simulink model "Q_CONTROL_Discret"  (Simulink 8.9)
settings: Solver=FixedStepDiscrete  StartTime=0.0  StopTime=inf  FixedStep=0.002  RelTol=1e-3  EnableMultiTasking=on
values from neighbouring files (symbols this model uses):
  K = place(AD,BD,pDisc)    [model3.m]
  Ts = results(i).Ts    [COMPLATE.m]    (also in model3.m = 0.002; observer_based-control.m = Ts_values(i))
undefined symbols (not defined in the file or in its folder): HIL, K_AMP, K_ENC, K_POT, qc_get_step_size, VMAX_AMP, VMAX_DAC
libraries: quarc_library x7, simulink_extras x4
settings Model: Creator=MLevis  LastModifiedBy=LEGION  SimulationMode=external  ExtModeTrigDuration=50000
settings SolverCC: PositivePriorityOrder=on
settings OptimizationCC: BooleanDataType=off  OptimizeBlockIOStorage=off  BufferReuse=off  GlobalBufferReuse=off  ExpressionFolding=off  ExpressionDepthLimit=2147483647  LocalBlockOutputs=off  InitFltsAndDblsToZero=on  LifeSpan=auto
settings DebuggingCC: SaveWithParameterizedLinksMsg=none  SignalResolutionControl=TryResolveAllWithWarning  MultiTaskDSMMsg=warning  MultiTaskCondExecSysMsg=none
settings RTWCC: Description=QUARC Win64 Target  SystemTargetFile=quarc_win64.tlc  TemplateMakefile=quarc_default_tmf
settings STFCustomTargetCC: TargetPreCompLibLocation=C:\PROGRA~3\QUARC\lib\2017a\win64\release  ConcurrentExecutionCompliant=on  SystemTargetFile=quarc_win64.tlc
settings GRTTargetCC: TargetPreCompLibLocation=C:\PROGRA~3\QUARC\lib\2017a\win64\release  ParMdlRefBuildCompliant=off  CompOptLevelCompliant=off  MatFileLogging=off  CPPClassGenCompliant=off  UseToolchainInfoCompliant=off  ExtMode=on  ExtModeMexFile=quarc_comm

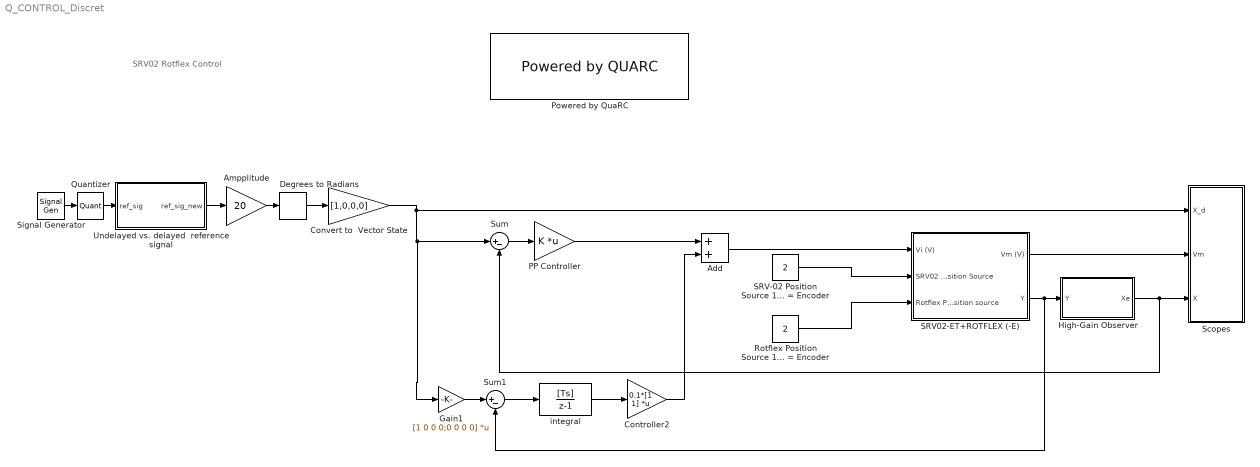
== system Q_CONTROL_Discret ==
  note: SRV02 Rotflex Control
  Add : Sum
  Ampplitude : Gain  Gain=20  SaturateOnIntegerOverflow=on  OutDataTypeStr=Inherit: Same as input  ParamDataTypeStr=Inherit: Same as input
  Controller2 : Gain  Gain=0.1*[1 1]  Multiplication=Matrix(K*u)  SaturateOnIntegerOverflow=on  OutDataTypeStr=Inherit: Same as input  ParamDataTypeStr=Inherit: Same as input
  Convert to  Vector State : Gain  Gain=[1,0,0,0]
  Degrees to Radians : simulink_extras/Transformations/Degrees to Radians
  Gain1 : Gain  Gain=[1 0 0 0;0 0 0 0]  Multiplication=Matrix(K*u)
  High-Gain Observer : Subsystem
  PP Controller : Gain  Gain=K  Multiplication=Matrix(K*u)  SaturateOnIntegerOverflow=on  OutDataTypeStr=Inherit: Same as input  ParamDataTypeStr=Inherit: Same as input
  Powered by QuaRC : quarc_library/Logos/Powered by QUARC
  Quantizer : Quantizer  QuantizationInterval=Ts
  "Rotflex Position Source 1 = Potentiometer, 2 = Encoder" : Constant  Value=2
  "SRV-02 Position Source 1 = Potentiometer, 2 = Encoder" : Constant  Value=2
  SRV02-ET+ROTFLEX (-E) : Subsystem
  Scopes : Subsystem
  Signal Generator : SignalGenerator  WaveForm=square  Frequency=0.3
  Sum : Sum  Inputs=|+-
  Sum1 : Sum  Inputs=|+-
  "Undelayed vs. delayed  reference signal " : Subsystem
  integral : DiscreteTransferFcn  Numerator=[Ts]  Denominator=[1 -1]  SampleTime=Ts
  wires:
  High-Gain Observer/1(Xe) -> Scopes/3(X), Sum/2
  SRV02-ET+ROTFLEX (-E)/2(Y) -> High-Gain Observer/1(Y), Sum1/2
  SRV02-ET+ROTFLEX (-E)/1(Vm (V)) -> Scopes/2(Vm)
  Sum/1 -> PP Controller/1
  Degrees to Radians/1 -> Convert to  Vector State/1
  Convert to  Vector State/1 -> Scopes/1(X_d), Gain1/1, Sum/1
  Ampplitude/1 -> Degrees to Radians/1
  Signal Generator/1 -> Quantizer/1
  "Undelayed vs. delayed  reference signal "/1(ref_sig_new) -> Ampplitude/1
  PP Controller/1 -> Add/1
  "SRV-02 Position Source 1 = Potentiometer, 2 = Encoder"/1 -> SRV02-ET+ROTFLEX (-E)/2(SRV02 Position Source)
  "Rotflex Position Source 1 = Potentiometer, 2 = Encoder"/1 -> SRV02-ET+ROTFLEX (-E)/3(Rotflex Position source)
  Quantizer/1 -> "Undelayed vs. delayed  reference signal "/1(ref_sig)
  Gain1/1 -> Sum1/1
  Sum1/1 -> integral/1
  integral/1 -> Controller2/1
  Add/1 -> SRV02-ET+ROTFLEX (-E)/1(Vi (V))
  Controller2/1 -> Add/2

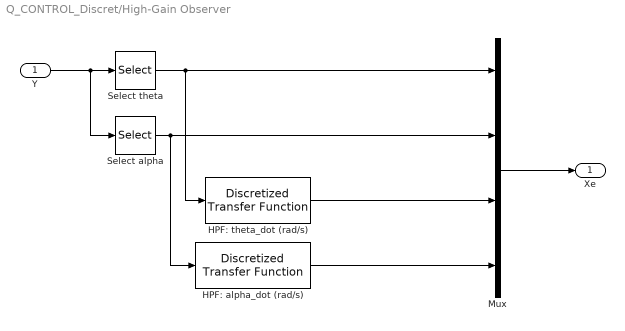
== system Q_CONTROL_Discret/High-Gain Observer ==
  Y : Inport  SampleTime=Ts
  HPF: alpha_dot (rad/s) : quarc_library/Discrete/Discretized Transfer Function  num=[150 0]  den=[1 150]  method=tustin  Ts=qc_get_step_size
  HPF: theta_dot (rad/s) : quarc_library/Discrete/Discretized Transfer Function  num=[150 0]  den=[1 150]  method=tustin  Ts=qc_get_step_size
  Mux : Mux
  Select alpha : Selector  InputPortWidth=2  IndexOptions=Index vector (dialog)  Indices=2  OutputSizes=1
  Select theta : Selector  InputPortWidth=2  IndexOptions=Index vector (dialog)  Indices=1  OutputSizes=1
  Xe : Outport  SampleTime=Ts
  wires:
  HPF: alpha_dot (rad/s)/1 -> Mux/4
  Select theta/1 -> HPF: theta_dot (rad/s)/1, Mux/1
  HPF: theta_dot (rad/s)/1 -> Mux/3
  Y/1 -> Select theta/1, Select alpha/1
  Mux/1 -> Xe/1
  Select alpha/1 -> HPF: alpha_dot (rad/s)/1, Mux/2

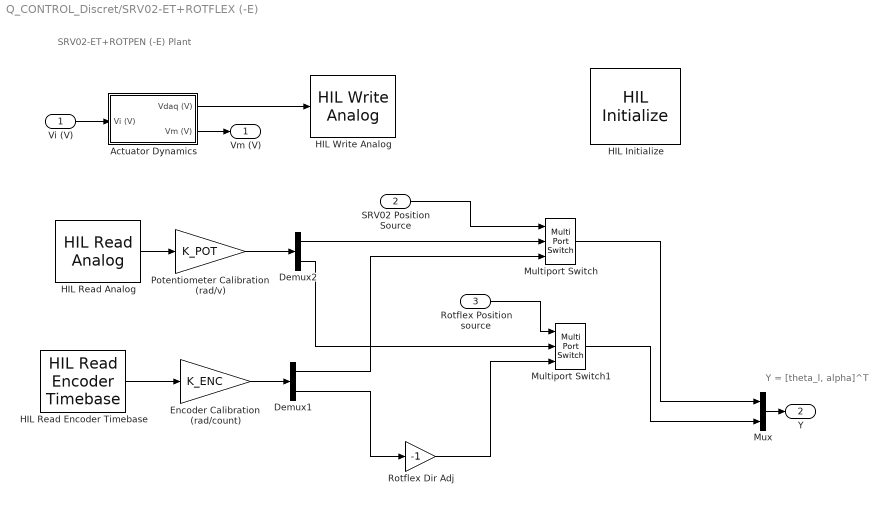
== system Q_CONTROL_Discret/SRV02-ET+ROTFLEX (-E) ==
  note: Y = [theta_l, alpha]^T
  note: SRV02-ET+ROTPEN (-E) Plant
  Vi (V) : Inport  SampleTime=Ts
  SRV02 Position Source : Inport  Port=2  SampleTime=Ts
  Rotflex Position source : Inport  Port=3  SampleTime=Ts
  Actuator Dynamics : Subsystem
  Demux1 : Demux  Outputs=2
  Demux2 : Demux  Outputs=2
  Encoder Calibration  (rad/count) : Gain  Gain=K_ENC  SaturateOnIntegerOverflow=on  OutDataTypeStr=Inherit: Same as input  ParamDataTypeStr=Inherit: Same as input
  HIL Initialize : quarc_library/Data Acquisition/Generic/Configuration/HIL Initialize  object_name=HIL-1  board_type=q2_usb  board_number=0  board_options=d0=digital;d1=digital;led=auto;update_rate=normal;decimation=1  exclusive=off  active=on  hardware_clocks=[0]  clock_modes=[]  initial_clock_frequencies=[]  set_clock_params_at_start=off  set_clock_params_at_switch_in=off  set_clock_frequencies_at_start=off  set_clock_frequencies_at_switch_in=off  analog_input_channels=[0:1]  analog_input_configurations=[]  analog_input_maximums=10  analog_input_minimums=-10  set_analog_input_params_at_start=on  set_analog_input_params_at_switch_in=off  analog_output_channels=[0:1]  analog_output_maximums=10  analog_output_minimums=-10  initial_analog_outputs=[0]  final_analog_outputs=[0]  watchdog_analog_outputs=0  set_analog_output_params_at_start=on  set_analog_output_params_at_switch_in=off  set_analog_outputs_at_start=on  set_analog_outputs_at_switch_in=off  set_analog_outputs_at_terminate=on  set_analog_outputs_at_switch_out=off  set_analog_outputs_on_watchdog=off  digital_input_channels=[]  digital_output_channels=[]  digital_output_configuration=[]  initial_digital_outputs=[1]  final_digital_outputs=[1]  watchdog_digital_outputs=[1]  set_digital_output_params_at_start=off  set_digital_output_params_at_switch_in=off  set_digital_outputs_at_start=on  set_digital_outputs_at_switch_in=off  set_digital_outputs_at_terminate=on  set_digital_outputs_at_switch_out=off  set_digital_outputs_on_watchdog=off  encoder_channels=[0:1]  quadrature=[4]  encoder_filter_frequency=[]  initial_encoder_counts=[0]  set_encoder_params_at_start=on  set_encoder_params_at_switch_in=off  set_encoder_counts_at_start=on  set_encoder_counts_at_switch_in=off  pwm_channels=[]  pwm_modes=[0]  pwm_frequency=1/0.020  pwm_configuration=[]  pwm_alignment=[]  pwm_polarity=[]  pwm_leading_deadband=[]  pwm_trailing_deadband=[]  initial_pwm_outputs=[0]  final_pwm_outputs=[0]  watchdog_pwm_outputs=[0]  set_pwm_params_at_start=on  set_pwm_params_at_switch_in=off  set_pwm_outputs_at_start=on  set_pwm_outputs_at_switch_in=off  set_pwm_outputs_at_terminate=on  set_pwm_outputs_at_switch_out=off  set_pwm_outputs_on_watchdog=off  other_output_channels=[]  initial_other_outputs=[]  final_other_outputs=[]  watchdog_other_outputs=[]  set_other_outputs_at_start=off  set_other_outputs_at_switch_in=off  set_other_outputs_at_terminate=off  set_other_outputs_at_switch_out=off  set_other_outputs_on_watchdog=off
      settings: AttributesFormatString=(%<object_name>)
  HIL Read Analog : quarc_library/Data Acquisition/Generic/Immediate I//O/HIL Read Analog  object_name=HIL-1  channels=0:1  sample_time=qc_get_step_size  active=on  vector_output=on
  HIL Read Encoder Timebase : quarc_library/Data Acquisition/Generic/Timebases/HIL Read Encoder Timebase  object_name=HIL-1  clock=0  channels=0:1  samples_in_buffer=max(ceil(1/qc_get_step_size), 1)  active=on  vector_output=on  data_type_mode=Inherit via back propagation  data_type=double
  HIL Write Analog : quarc_library/Data Acquisition/Generic/Immediate I//O/HIL Write Analog  object_name=HIL-1  channels=0  sample_time=-1  active=off  vector_input=off
  Multiport Switch : MultiPortSwitch  Inputs=2
  Multiport Switch1 : MultiPortSwitch  Inputs=2
  Mux : Mux  Inputs=2
  Potentiometer Calibration  (rad/v) : Gain  Gain=K_POT  SaturateOnIntegerOverflow=on  OutDataTypeStr=Inherit: Same as input  ParamDataTypeStr=Inherit: Same as input
  Rotflex Dir Adj : Gain  Gain=-1
  Vm (V) : Outport  SampleTime=Ts  InitialOutput=0
  Y : Outport  Port=2  SampleTime=Ts  InitialOutput=0
  wires:
  Demux1/2 -> Rotflex Dir Adj/1
  Mux/1 -> Y/1
  Vi (V)/1 -> Actuator Dynamics/1(Vi (V))
  Actuator Dynamics/1(Vdaq (V)) -> HIL Write Analog/1
  Actuator Dynamics/2(Vm (V)) -> Vm (V)/1
  Encoder Calibration  (rad/count)/1 -> Demux1/1
  HIL Read Encoder Timebase/1 -> Encoder Calibration  (rad/count)/1
  HIL Read Analog/1 -> Potentiometer Calibration  (rad/v)/1
  Multiport Switch/1 -> Mux/1
  SRV02 Position Source/1 -> Multiport Switch/1
  Rotflex Dir Adj/1 -> Multiport Switch1/3
  Potentiometer Calibration  (rad/v)/1 -> Demux2/1
  Demux2/1 -> Multiport Switch/2
  Demux1/1 -> Multiport Switch/3
  Rotflex Position source/1 -> Multiport Switch1/1
  Multiport Switch1/1 -> Mux/2
  Demux2/2 -> Multiport Switch1/2

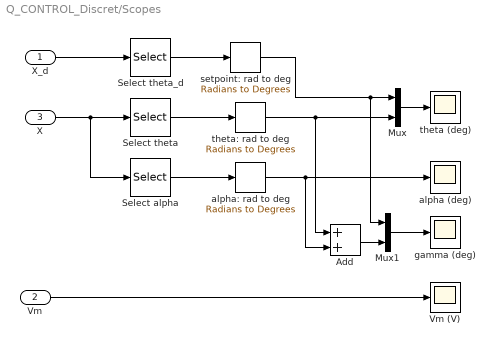
== system Q_CONTROL_Discret/Scopes ==
  X_d : Inport  SampleTime=Ts
  Vm : Inport  Port=2  SampleTime=Ts
  X : Inport  Port=3  SampleTime=Ts
  Add : Sum
  Mux : Mux  Inputs=2
  Mux1 : Mux  Inputs=2
  Select alpha : Selector  InputPortWidth=4  IndexOptions=Index vector (dialog)  Indices=2  OutputSizes=1
  Select theta : Selector  InputPortWidth=4  IndexOptions=Index vector (dialog)  Indices=1  OutputSizes=1
  Select theta_d : Selector  InputPortWidth=4  IndexOptions=Index vector (dialog)  Indices=1  OutputSizes=1
  Vm (V) : Scope
  alpha (deg) : Scope
  alpha: rad to deg : simulink_extras/Transformations/Radians to Degrees
  gamma (deg) : Scope
  setpoint: rad to deg : simulink_extras/Transformations/Radians to Degrees
  theta (deg) : Scope
  theta: rad to deg : simulink_extras/Transformations/Radians to Degrees
  wires:
  Select theta_d/1 -> setpoint: rad to deg/1
  setpoint: rad to deg/1 -> Mux/1, Mux1/1
  X/1 -> Select theta/1, Select alpha/1
  alpha: rad to deg/1 -> alpha (deg)/1, Add/2
  Select theta/1 -> theta: rad to deg/1
  Select alpha/1 -> alpha: rad to deg/1
  theta: rad to deg/1 -> Mux/2, Add/1
  Mux/1 -> theta (deg)/1
  X_d/1 -> Select theta_d/1
  Vm/1 -> Vm (V)/1
  Add/1 -> Mux1/2
  Mux1/1 -> gamma (deg)/1

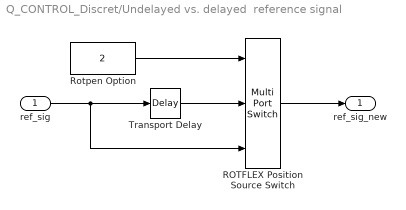
== system Q_CONTROL_Discret/Undelayed vs. delayed  reference signal  ==
  ref_sig : Inport  SampleTime=Ts
  ROTFLEX Position Source Switch : MultiPortSwitch  DataPortOrder=Zero-based contiguous  Inputs=2  zeroidx=on
  Rotpen Option : Constant  Value=2  SampleTime=Ts
  Transport Delay : TransportDelay  DelayTime=0.1
  ref_sig_new : Outport  SampleTime=Ts
  wires:
  Rotpen Option/1 -> ROTFLEX Position Source Switch/1
  ref_sig/1 -> ROTFLEX Position Source Switch/3, Transport Delay/1
  Transport Delay/1 -> ROTFLEX Position Source Switch/2
  ROTFLEX Position Source Switch/1 -> ref_sig_new/1

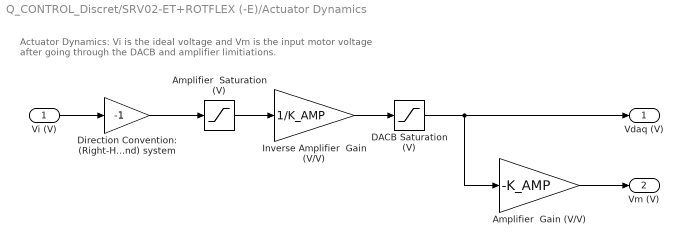
== system Q_CONTROL_Discret/SRV02-ET+ROTFLEX (-E)/Actuator Dynamics ==
  note: Actuator Dynamics: Vi is the ideal voltage and Vm is the
      | input motor voltage after going through the DACB and amplifier limitiations.
  Vi (V) : Inport  SampleTime=Ts
  Amplifier  Gain (V/V) : Gain  Gain=-K_AMP
  Amplifier  Saturation (V) : Saturate  UpperLimit=VMAX_AMP  LowerLimit=-VMAX_AMP
  DACB Saturation (V) : Saturate  UpperLimit=VMAX_DAC  LowerLimit=-VMAX_DAC
  Direction Convention: (Right-Hand) system : Gain  Gain=-1  SaturateOnIntegerOverflow=on  OutDataTypeStr=Inherit: Same as input  ParamDataTypeStr=Inherit: Same as input
  Inverse Amplifier  Gain (V/V) : Gain  Gain=1/K_AMP
  Vdaq (V) : Outport  SampleTime=Ts
  Vm (V) : Outport  Port=2  SampleTime=Ts
  wires:
  Vi (V)/1 -> Direction Convention: (Right-Hand) system/1
  Amplifier  Saturation (V)/1 -> Inverse Amplifier  Gain (V/V)/1
  Inverse Amplifier  Gain (V/V)/1 -> DACB Saturation (V)/1
  DACB Saturation (V)/1 -> Amplifier  Gain (V/V)/1, Vdaq (V)/1
  Amplifier  Gain (V/V)/1 -> Vm (V)/1
  Direction Convention: (Right-Hand) system/1 -> Amplifier  Saturation (V)/1
